simulink subsystem "reutrn_water_controller"  (R2022b)
settings: Solver=VariableStepAuto  StartTime=0.0  StopTime=inf  RelTol=1e-3
model mask{tank_pump_max=530, consumer_min=150, consumer_max=500, switch_time=60, tank_pump_ref=300}
  mask prompts: tank_pump_max "Tank pump max [mm]"; consumer_min "Tank consumer min [mm]"; consumer_max "Tank consumer max [mm]"; switch_time "Aux pump switch time [s]"; tank_pump_ref "Tank pump ref [mm]"
libraries: simulink x3
settings Model: DefaultTestHarness=reutrn_water_controller_Harness1  Creator=laula  LastModifiedBy=laula

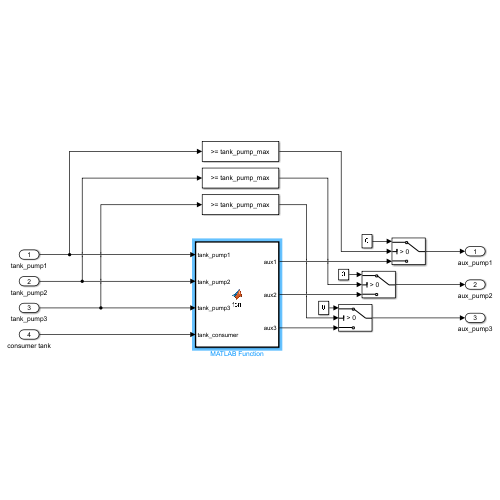
[thumbnail: Simulink's stored preview of the top-level diagram]
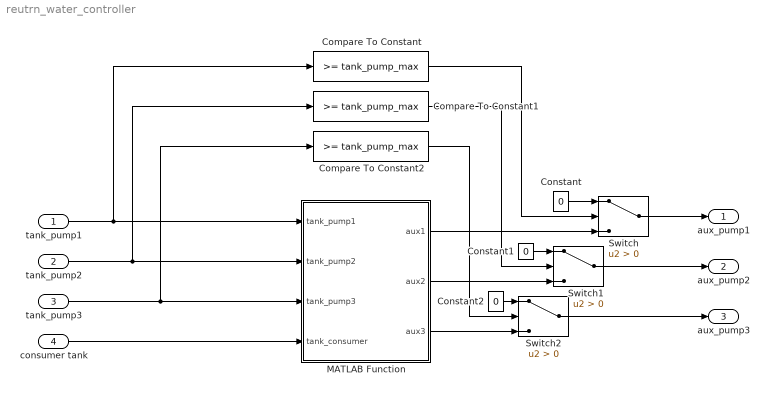
== system reutrn_water_controller ==
  tank_pump1 : Inport
  tank_pump2 : Inport  Port=2
  tank_pump3 : Inport  Port=3
  consumer tank : Inport  Port=4
  Compare To Constant : simulink/Logic and Bit Operations/Compare To Constant  relop=>=  const=tank_pump_max  OutDataTypeStr=boolean
  Compare To Constant1 : simulink/Logic and Bit Operations/Compare To Constant  relop=>=  const=tank_pump_max  OutDataTypeStr=boolean
  Compare To Constant2 : simulink/Logic and Bit Operations/Compare To Constant  relop=>=  const=tank_pump_max  OutDataTypeStr=boolean
  Constant : Constant  Value=0
  Constant1 : Constant  Value=0
  Constant2 : Constant  Value=0
  MATLAB Function : MATLAB Function  TreatAsAtomicUnit=on  SystemSampleTime=1
  Switch : Switch  Criteria=u2 > Threshold  SaturateOnIntegerOverflow=off  InputSameDT=off
  Switch1 : Switch  Criteria=u2 > Threshold  SaturateOnIntegerOverflow=off  InputSameDT=off
  Switch2 : Switch  Criteria=u2 > Threshold  SaturateOnIntegerOverflow=off  InputSameDT=off
  aux_pump1 : Outport
  aux_pump2 : Outport  Port=2
  aux_pump3 : Outport  Port=3
  wires:
  tank_pump1/1 -> Compare To Constant/1, MATLAB Function/1(tank_pump1)
  tank_pump2/1 -> Compare To Constant1/1, MATLAB Function/2(tank_pump2)
  tank_pump3/1 -> Compare To Constant2/1, MATLAB Function/3(tank_pump3)
  consumer tank/1 -> MATLAB Function/4(tank_consumer)
  MATLAB Function/1(aux1) -> Switch/3
  MATLAB Function/2(aux2) -> Switch1/3
  MATLAB Function/3(aux3) -> Switch2/3
  Compare To Constant/1 -> Switch/2
  Compare To Constant1/1 -> Switch1/2
  Compare To Constant2/1 -> Switch2/2
  Constant/1 -> Switch/1
  Constant1/1 -> Switch1/1
  Constant2/1 -> Switch2/1
  Switch/1 -> aux_pump1/1
  Switch1/1 -> aux_pump2/1
  Switch2/1 -> aux_pump3/1

== matlab function reutrn_water_controller/MATLAB Function ==
  data: tank_pump1 input; aux1 output; tank_pump2 input; tank_pump3 input; tank_consumer input; aux2 output; aux3 output; consumer_min parameter; consumer_max parameter; switch_time parameter; tank_pump_ref parameter
function [aux1, aux2, aux3] = fcn(tank_pump1, tank_pump2, tank_pump3, tank_consumer, consumer_min, consumer_max, switch_time, tank_pump_ref)
%Function to be called every second
persistent time_since_switch
if(isempty(time_since_switch)); time_since_switch = 0; end 
persistent index 
if(isempty(index)); index = 1; end

time_since_switch = time_since_switch + 1;

aux1 = 0;
aux2 = 0;
aux3 = 0;

if(tank_consumer>consumer_max)
    aux1 = 100;
    aux2 = 100;
    aux3 = 100;
    return
elseif(tank_consumer<consumer_min)
    aux1 = 0;
    aux2 = 0;
    aux3 = 0;
    return
elseif(min([tank_pump1, tank_pump2, tank_pump3]) < tank_pump_ref)
    if(time_since_switch>switch_time)
        time_since_switch = 0;
        [~,index] = min([tank_pump1, tank_pump2, tank_pump3]);
    end
    switch index
        case 1
            aux1 = 100;
        case 2
            aux2 = 100;
        case 3
            aux3 = 100;
    end
    
end
